simulink model "Antriebsstrangmodell_V2"  (R2019a)
settings: Solver=FixedStepAuto  StartTime=0.0  StopTime=t_Simulation  FixedStep=dt  RelTol=1e-3
undefined symbols (not defined in the file): alpha_Rotor, alpha_Stator, Anteil_Stator, cp_Luft, D_2a, delta, eta_EMaschine_Break_M_EMaschine, eta_EMaschine_Break_M_EMaschine_reku, eta_EMaschine_Break_n_EMaschine, eta_EMaschine_Break_n_EMaschine_reku, eta_EMaschine_Faktor_Volllast, eta_EMaschine_Table, eta_EMaschine_Table_reku, h_WC_pumpoff, h_WC_pumpon, lam_Luft, M_EMaschine_max, m_ER, m_RSL, m_RTO, m_RYO, m_SSL, m_STO, m_SYO, m_WH, nue_Luft, pump_start_limit, rho_Luft, share_EMaschine_Ummagnet_reku_Table, share_EMaschine_Ummagnet_Table, share_EMaschine_Wicklung_reku_Table, share_EMaschine_Wicklung_Table, share_EMaschine_WirkMech_reku_Table, share_EMaschine_WirkMech_Table, share_EMaschine_WirkZus_reku_Table, share_EMaschine_WirkZus_Table, T_Entwurf_Rotor, T_Entwurf_Stator, t_Simulation, T_Start_EMaschine, v_EC_corr, v_ER_corr, v_WH_corr, Verlustleistung_Fit
libraries: fl_lib x72, nesl_utility x26, SimscapeCustomBlocks_lib x8, simulink x3
(part 1 of 2)
settings Model: Creator=Ludwig Stolle  LastModifiedBy=Ludwig Stolle
settings DataIOCC: SaveOutput=off  SignalLogging=off  DSMLogging=off  SaveTime=off  ReturnWorkspaceOutputs=off
settings DebuggingCC: UnconnectedInputMsg=none  UnconnectedOutputMsg=none

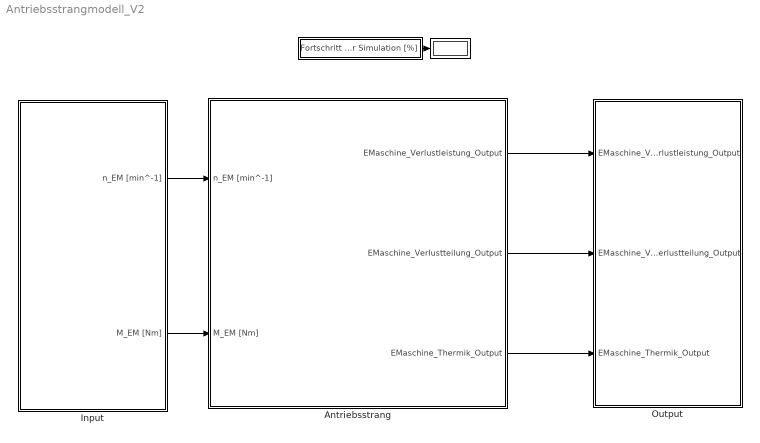
== system Antriebsstrangmodell_V2 ==
  "\t\t     " : Subsystem
  " " : Display
      settings: Format=bank
  Antriebsstrang : Subsystem
  Input : Subsystem
  Output : Subsystem
  wires:
  Input/1(n_EM [min^-1]) -> Antriebsstrang/1(n_EM [min^-1])
  Input/2(M_EM [Nm]) -> Antriebsstrang/2(M_EM [Nm])
  "\t\t     "/1(Fortschritt der Simulation [%]) -> " "/1
  Antriebsstrang/1(EMaschine_Verlustleistung_Output) -> Output/1(EMaschine_Verlustleistung_Output)
  Antriebsstrang/2(EMaschine_Verlustteilung_Output) -> Output/2(EMaschine_Verlustteilung_Output)
  Antriebsstrang/3(EMaschine_Thermik_Output) -> Output/3(EMaschine_Thermik_Output)

== system Antriebsstrangmodell_V2/		      ==
  note: Fortschritt der Simulation = 100 * simulierte Zeit / t_Simulation
      |
      | mit Fortschritt der Simulation in %
  Clock : Clock
  Constant : Constant  Value=t_Simulation  VectorParams1D=off
  Divide : Product  Inputs=*/
  Umrechnung in % : Gain  Gain=100
  Fortschritt der Simulation [%] : Outport
  wires:
  Constant/1 -> Divide/2
  Clock/1 -> Divide/1
  Divide/1 -> Umrechnung in %/1
  Umrechnung in %/1 -> Fortschritt der Simulation [%]/1

== system Antriebsstrangmodell_V2/Antriebsstrang ==
  n_EM [min^-1] : Inport
  M_EM [Nm] : Inport  Port=2
  E-Maschine Thermik : Subsystem
  E-Maschine Verlustleistung : Subsystem
  E-Maschine Verlustteilung : Subsystem
  EMaschine_Verlustleistung_Output : Outport
  EMaschine_Verlustteilung_Output : Outport  Port=2
  EMaschine_Thermik_Output : Outport  Port=3
  wires:
  M_EM [Nm]/1 -> E-Maschine Verlustteilung/3(M_EM [Nm]), E-Maschine Verlustleistung/2(M_EM [Nm])
  n_EM [min^-1]/1 -> E-Maschine Thermik/2(n_EM [min^-1]), E-Maschine Verlustteilung/2(n_EM [min^-1]), E-Maschine Verlustleistung/1(n_EM [min^-1])
  E-Maschine Verlustleistung/1(EMaschine_Verlustleistung_Output) -> EMaschine_Verlustleistung_Output/1, E-Maschine Verlustteilung/1(EMaschine_Verlustleistung_Output)
  E-Maschine Verlustteilung/1(EMaschine_Verlustteilung_Output) -> EMaschine_Verlustteilung_Output/1, E-Maschine Thermik/1(EMaschine_Verlustlteilung_Output)
  E-Maschine Thermik/1(EMaschine_Thermik_Output) -> EMaschine_Thermik_Output/1

== system Antriebsstrangmodell_V2/Input ==
  From Workspace : FromWorkspace  VariableName=n_EM  SampleTime=0  OutputAfterFinalValue=Setting to zero
  From Workspace1 : FromWorkspace  VariableName=M_EM  SampleTime=0  OutputAfterFinalValue=Setting to zero
  Product : Product
  Ramp : simulink/Sources/Ramp  slope=0.05  start=0  InitialOutput=0
  Saturation : Saturate  UpperLimit=1  LowerLimit=0
  n_EM [min^-1] : Outport
  M_EM [Nm] : Outport  Port=2
  wires:
  From Workspace/1 -> n_EM [min^-1]/1
  Saturation/1 -> Product/2
  From Workspace1/1 -> Product/1
  Product/1 -> M_EM [Nm]/1
  Ramp/1 -> Saturation/1

== system Antriebsstrangmodell_V2/Output ==
  note: -> Die Simulationsergebnisse, die an MATLAB übergeben werden sollen, müssen einkommentiert sein
      | -> Falls bestimmte Simualtionsergebnisse nicht an MATLAB übergeben werden sollen, dann müssen diese auskommentiert werden
  EMaschine_Verlustleistung_Output : Inport
  EMaschine_Verlustteilung_Output : Inport  Port=2
  EMaschine_Thermik_Output : Inport  Port=3
  E-Maschine Thermik : ToWorkspace  VariableName=EMaschine_Thermik_Output  SaveFormat=Timeseries  SampleTime=-1
      settings: Decimation=Decimation_Output
  E-Maschine Verlustleistung : ToWorkspace  VariableName=EMaschine_Verlustleistung_Output  SaveFormat=Timeseries  SampleTime=-1
      settings: Decimation=Decimation_Output
  E-Maschine Verlustteilung : ToWorkspace  VariableName=EMaschine_Verlustteilung_Output  SaveFormat=Timeseries  SampleTime=-1
      settings: Decimation=Decimation_Output
  wires:
  EMaschine_Verlustleistung_Output/1 -> E-Maschine Verlustleistung/1
  EMaschine_Verlustteilung_Output/1 -> E-Maschine Verlustteilung/1
  EMaschine_Thermik_Output/1 -> E-Maschine Thermik/1

== system Antriebsstrangmodell_V2/Antriebsstrang/E-Maschine Thermik ==
  EMaschine_Verlustlteilung_Output : Inport
  n_EM [min^-1] : Inport  Port=2
  Aufteilung mechanischer Verluste : Subsystem
  Bus Creator : BusCreator  Inputs=5
  Bus Selector1 : BusSelector  OutputSignals=P_Verlust_EMaschine_Wicklung [W],P_Verlust_EMaschine_Ummagnet [W],P_Verlust_EMaschine_WirkZus [W],P_Verlust_EMaschine_WirkMech [W]
  Thermisches Netzwerk1 : Subsystem
  Wärmeübergangskoeffizienten Konvektion Luftspalt und Endcap-Luft : Subsystem
  EMaschine_Thermik_Output : Outport
  wires:
  EMaschine_Verlustlteilung_Output/1 -> Bus Selector1/1
  Bus Creator/1 -> EMaschine_Thermik_Output/1
  Bus Selector1/2 -> Thermisches Netzwerk1/2(P_Verlust_EMaschine_Ummagnet [W])  "<P_Verlust_EMaschine_Ummagnet [W]>"
  Bus Selector1/3 -> Thermisches Netzwerk1/3(P_Verlust_EMaschine_WirkZus [W])  "<P_Verlust_EMaschine_WirkZus [W]>"
  Bus Selector1/1 -> Thermisches Netzwerk1/1(P_Verlust_EMaschine_Wicklung [W])  "<P_Verlust_EMaschine_Wicklung [W]>"
  Wärmeübergangskoeffizienten Konvektion Luftspalt und Endcap-Luft/1(HTC_Luftspalt [W*m^-2*K^-1]) -> Thermisches Netzwerk1/6(HTC_Luftspalt [W*m^-2*K^-1])  "HTC_Luftspalt [W*m^-2*K^-1]"
  Wärmeübergangskoeffizienten Konvektion Luftspalt und Endcap-Luft/2(HTC_Endcap [W*m^-2*K^-1]) -> Thermisches Netzwerk1/7(HTC_Endcap [W*m^-2*K^-1])  "HTC_Endcap [W*m^-2*K^-1]"
  Wärmeübergangskoeffizienten Konvektion Luftspalt und Endcap-Luft/3(HTC_Kurzschlussring [W*m^-2*K^-1]) -> Thermisches Netzwerk1/8(HTC_Kurzschlussring [W*m^-2*K^-1])  "HTC_Kurzschlussring [W*m^-2*K^-1]"
  Wärmeübergangskoeffizienten Konvektion Luftspalt und Endcap-Luft/4(HTC_Wickelkopf [W*m^-2*K^-1]) -> Thermisches Netzwerk1/9(HTC_Wickelkopf [W*m^-2*K^-1])  "HTC_Wickelkopf [W*m^-2*K^-1]"
  Aufteilung mechanischer Verluste/1(P_Verlust_EMaschine_Luftwiderstand [W]) -> Thermisches Netzwerk1/4(P_Verlust_EMaschine_Luftwiderstand [W])
  Bus Selector1/4 -> Aufteilung mechanischer Verluste/1(P_Verlust_EMaschine_WirkMech [W])  "<P_Verlust_EMaschine_WirkMech [W]>"
  Aufteilung mechanischer Verluste/2(P_Verlust_EMaschine_Lager [W]) -> Thermisches Netzwerk1/5(P_Verlust_EMaschine_Lager [W])
  Thermisches Netzwerk1/1(T_EMaschine_Wickelkopf [K]) -> Bus Creator/1
  Thermisches Netzwerk1/2(T_EMaschine_Kuehlmittel [K]) -> Bus Creator/2
  n_EM [min^-1]/1 -> Aufteilung mechanischer Verluste/2(n_EMaschine [min^-1]), Wärmeübergangskoeffizienten Konvektion Luftspalt und Endcap-Luft/1(<n_EMaschine [min^-1]>)
  Thermisches Netzwerk1/4(T_EMaschine_Kurzschlussring [K]) -> Bus Creator/4
  Thermisches Netzwerk1/5(T_EMaschine_Rotorstaebe [K]) -> Bus Creator/5
  Thermisches Netzwerk1/3(T_EMaschine_Wicklung [K]) -> Bus Creator/3

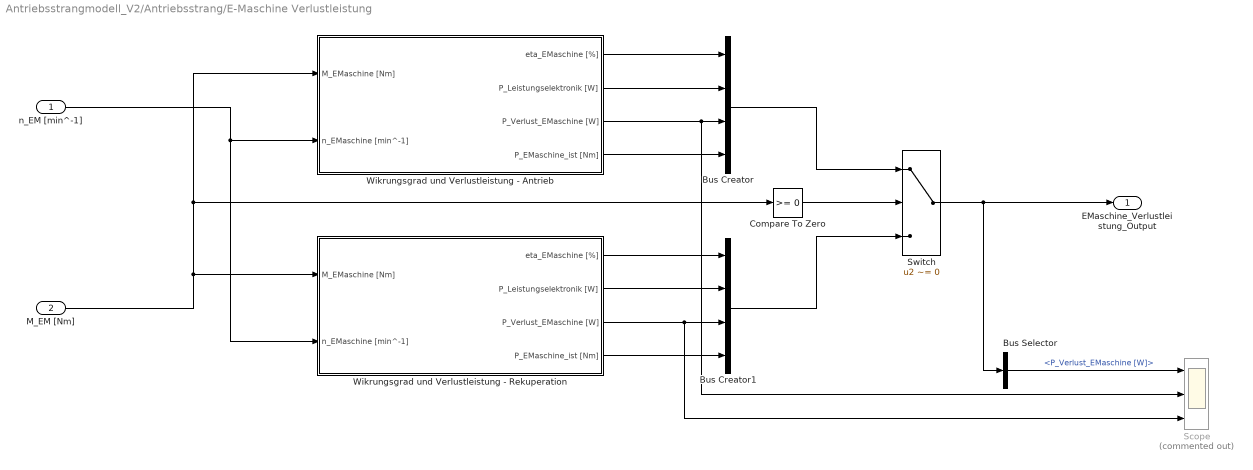
== system Antriebsstrangmodell_V2/Antriebsstrang/E-Maschine Verlustleistung ==
  n_EM [min^-1] : Inport
  M_EM [Nm] : Inport  Port=2
  Bus Creator : BusCreator  Inputs=4
  Bus Creator1 : BusCreator  Inputs=4
  Bus Selector : BusSelector  OutputSignals=P_Verlust_EMaschine [W]
  Compare To Zero : simulink/Logic and Bit Operations/Compare To Zero  relop=>=  OutDataTypeStr=boolean
  Scope : Scope  Commented=on  NumInputPorts=3
  Switch : Switch  Criteria=u2 ~= 0
  Wikrungsgrad und Verlustleistung - Antrieb : Subsystem
  Wikrungsgrad und Verlustleistung - Rekuperation : Subsystem
  EMaschine_Verlustleistung_Output : Outport
  wires:
  Wikrungsgrad und Verlustleistung - Antrieb/1(eta_EMaschine [%]) -> Bus Creator/1
  Wikrungsgrad und Verlustleistung - Antrieb/2(P_Leistungselektronik [W]) -> Bus Creator/2
  Wikrungsgrad und Verlustleistung - Antrieb/3(P_Verlust_EMaschine [W]) -> Scope/2, Bus Creator/3
  Wikrungsgrad und Verlustleistung - Rekuperation/1(eta_EMaschine [%]) -> Bus Creator1/1
  Wikrungsgrad und Verlustleistung - Rekuperation/2(P_Leistungselektronik [W]) -> Bus Creator1/2
  Wikrungsgrad und Verlustleistung - Rekuperation/3(P_Verlust_EMaschine [W]) -> Scope/3, Bus Creator1/3
  Bus Creator/1 -> Switch/1
  Bus Creator1/1 -> Switch/3
  Compare To Zero/1 -> Switch/2
  Switch/1 -> Bus Selector/1, EMaschine_Verlustleistung_Output/1
  Bus Selector/1 -> Scope/1  "<P_Verlust_EMaschine [W]>"
  Wikrungsgrad und Verlustleistung - Antrieb/4(P_EMaschine_ist [Nm]) -> Bus Creator/4
  Wikrungsgrad und Verlustleistung - Rekuperation/4(P_EMaschine_ist [Nm]) -> Bus Creator1/4
  n_EM [min^-1]/1 -> Wikrungsgrad und Verlustleistung - Rekuperation/2(n_EMaschine [min^-1]), Wikrungsgrad und Verlustleistung - Antrieb/2(n_EMaschine [min^-1])
  M_EM [Nm]/1 -> Wikrungsgrad und Verlustleistung - Antrieb/1(M_EMaschine [Nm]), Compare To Zero/1, Wikrungsgrad und Verlustleistung - Rekuperation/1(M_EMaschine [Nm])

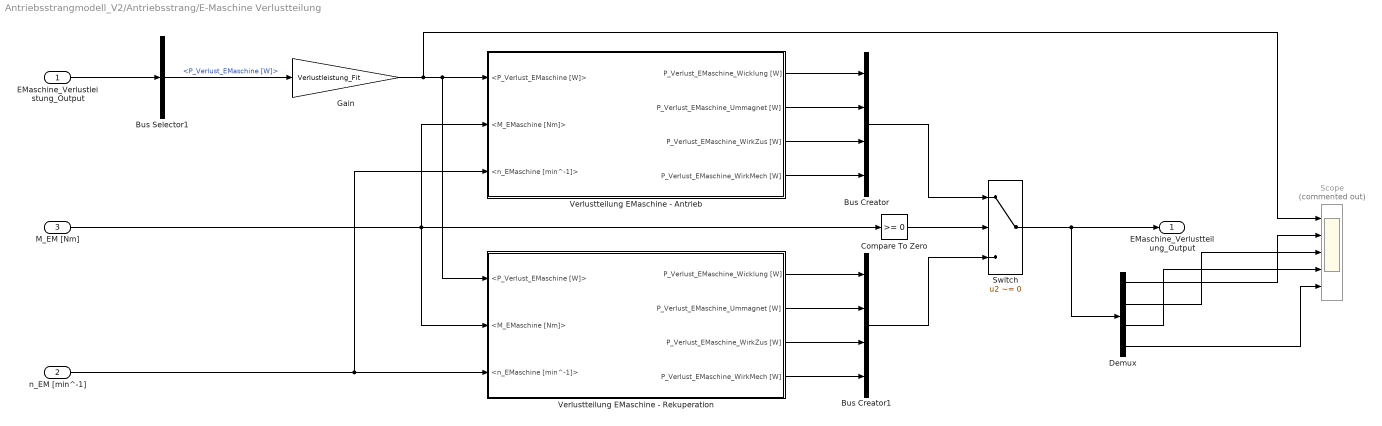
== system Antriebsstrangmodell_V2/Antriebsstrang/E-Maschine Verlustteilung ==
  EMaschine_Verlustleistung_Output : Inport
  n_EM [min^-1] : Inport  Port=2
  M_EM [Nm] : Inport  Port=3
  Bus Creator : BusCreator  Inputs=4
  Bus Creator1 : BusCreator  Inputs=4
  Bus Selector1 : BusSelector  OutputSignals=P_Verlust_EMaschine [W]
  Compare To Zero : simulink/Logic and Bit Operations/Compare To Zero  relop=>=  OutDataTypeStr=boolean
  Demux : Demux
  Gain : Gain  Gain=Verlustleistung_Fit
  Scope : Scope  Commented=on  NumInputPorts=5
  Switch : Switch  Criteria=u2 ~= 0
  Verlustteilung EMaschine - Antrieb : Subsystem
  Verlustteilung EMaschine - Rekuperation : Subsystem
  EMaschine_Verlustteilung_Output : Outport
  wires:
  EMaschine_Verlustleistung_Output/1 -> Bus Selector1/1
  Bus Selector1/1 -> Gain/1  "<P_Verlust_EMaschine [W]>"
  Verlustteilung EMaschine - Antrieb/1(P_Verlust_EMaschine_Wicklung [W]) -> Bus Creator/1
  Verlustteilung EMaschine - Antrieb/2(P_Verlust_EMaschine_Ummagnet [W]) -> Bus Creator/2
  Verlustteilung EMaschine - Antrieb/3(P_Verlust_EMaschine_WirkZus [W]) -> Bus Creator/3
  Verlustteilung EMaschine - Antrieb/4(P_Verlust_EMaschine_WirkMech [W]) -> Bus Creator/4
  Compare To Zero/1 -> Switch/2
  Switch/1 -> Demux/1, EMaschine_Verlustteilung_Output/1
  Bus Creator/1 -> Switch/1
  Verlustteilung EMaschine - Rekuperation/1(P_Verlust_EMaschine_Wicklung [W]) -> Bus Creator1/1
  Verlustteilung EMaschine - Rekuperation/2(P_Verlust_EMaschine_Ummagnet [W]) -> Bus Creator1/2
  Verlustteilung EMaschine - Rekuperation/3(P_Verlust_EMaschine_WirkZus [W]) -> Bus Creator1/3
  Verlustteilung EMaschine - Rekuperation/4(P_Verlust_EMaschine_WirkMech [W]) -> Bus Creator1/4
  Bus Creator1/1 -> Switch/3
  Gain/1 -> Scope/1, Verlustteilung EMaschine - Rekuperation/1(<P_Verlust_EMaschine [W]>), Verlustteilung EMaschine - Antrieb/1(<P_Verlust_EMaschine [W]>)
  Demux/4 -> Scope/5
  Demux/1 -> Scope/2
  Demux/2 -> Scope/3
  Demux/3 -> Scope/4
  n_EM [min^-1]/1 -> Verlustteilung EMaschine - Antrieb/3(<n_EMaschine [min^-1]>), Verlustteilung EMaschine - Rekuperation/3(<n_EMaschine [min^-1]>)
  M_EM [Nm]/1 -> Verlustteilung EMaschine - Rekuperation/2(<M_EMaschine [Nm]>), Verlustteilung EMaschine - Antrieb/2(<M_EMaschine [Nm]>), Compare To Zero/1

== system Antriebsstrangmodell_V2/Antriebsstrang/E-Maschine Thermik/Aufteilung mechanischer Verluste ==
  note: Berechnung der Anteile von Luftwiderstand und Lagerverlusten an ges. mechanischem Verlust nach CHIN 2018.
      | Verluste sind nur von der Drehzahl abhängig. Daher normierte Verluste angenähert mittels Polynom 2. Grades für Luftwiderstand
      | und Polynom 1. Grades für Lagerreibung.
  P_Verlust_EMaschine_WirkMech [W] : Inport
  n_EMaschine [min^-1] : Inport  Port=2
  Abs : Abs
  Add : Sum
  Add1 : Sum  Inputs=+-
  Divide : Product  Inputs=/*
  Divide1 : Product  Inputs=**
  Polynomial : Polyval  Coefs=[+0.0026e-5, -0.25e-5, 0]
  Polynomial1 : Polyval  Coefs=[+0.06e-3, +0.05]
  P_Verlust_EMaschine_Luftwiderstand [W] : Outport
  P_Verlust_EMaschine_Lager [W] : Outport  Port=2
  wires:
  n_EMaschine [min^-1]/1 -> Abs/1
  Abs/1 -> Polynomial1/1, Polynomial/1
  Polynomial1/1 -> Divide/2, Add/2  "Normierter Lagerverlust"
  Polynomial/1 -> Add/1  "Normierte Luftreibung"
  Add/1 -> Divide/1
  P_Verlust_EMaschine_WirkMech [W]/1 -> Add1/1, Divide1/1
  Divide/1 -> Divide1/2  "Anteil Lagerverluste am gesamten mechanischen Verlust"
  Divide1/1 -> Add1/2, P_Verlust_EMaschine_Lager [W]/1  "P_Verlust_EMaschine_Lager [W]"
  Add1/1 -> P_Verlust_EMaschine_Luftwiderstand [W]/1  "P_Verlust_EMaschine_Luftwiderstand [W]"

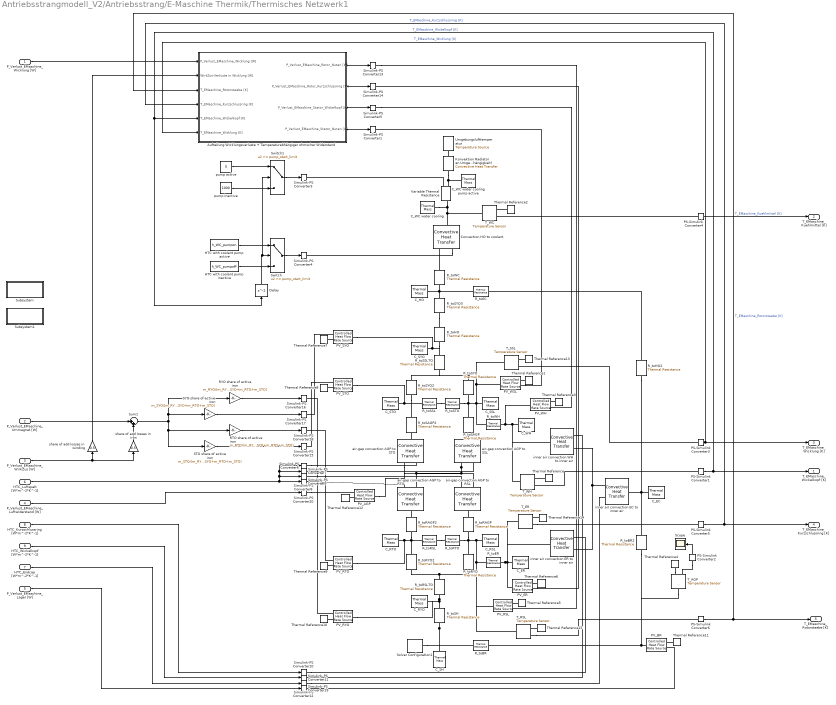
== system Antriebsstrangmodell_V2/Antriebsstrang/E-Maschine Thermik/Thermisches Netzwerk1 ==
  P_Verlust_EMaschine_Wicklung [W] : Inport
  P_Verlust_EMaschine_Ummagnet [W] : Inport  Port=2
  P_Verlust_EMaschine_WirkZus [W] : Inport  Port=3
  P_Verlust_EMaschine_Luftwiderstand [W] : Inport  Port=4
  P_Verlust_EMaschine_Lager [W] : Inport  Port=5
  HTC_Luftspalt [W*m^-2*K^-1] : Inport  Port=6
  HTC_Endcap [W*m^-2*K^-1] : Inport  Port=7
  HTC_Kurzschlussring [W*m^-2*K^-1] : Inport  Port=8
  HTC_Wickelkopf [W*m^-2*K^-1] : Inport  Port=9
  Aufteilung Wicklungsverluste + Temperaturabhängiger ohmscher Widerstand : Subsystem
  C_EC : fl_lib/Thermal/Thermal Elements/Thermal Mass  mass=m_EC kg  sp_heat=cp_EC J/kg/K  T_specify=on  T_priority=High  T=T_Start_EMaschine K  T_nominal_specify=off  T_nominal_unit=K  T_nominal_value=1  Q_specify=off  Q_priority=None  Q=0 W  Q_nominal_specify=off  Q_nominal_unit=W  Q_nominal_value=1
  C_ER : fl_lib/Thermal/Thermal Elements/Thermal Mass  mass=m_ER kg  sp_heat=cp_ER J/kg/K  T_specify=on  T_priority=High  T=T_Start_EMaschine K  T_nominal_specify=off  T_nominal_unit=K  T_nominal_value=1  Q_specify=off  Q_priority=None  Q=0 W  Q_nominal_specify=off  Q_nominal_unit=W  Q_nominal_value=1
  C_HO : fl_lib/Thermal/Thermal Elements/Thermal Mass  mass=m_HO kg  sp_heat=cp_HO J/kg/K  T_specify=on  T_priority=High  T=T_Start_EMaschine K  T_nominal_specify=off  T_nominal_unit=K  T_nominal_value=1  Q_specify=off  Q_priority=None  Q=0 W  Q_nominal_specify=off  Q_nominal_unit=W  Q_nominal_value=1
  C_RSL : fl_lib/Thermal/Thermal Elements/Thermal Mass  mass=m_RSL kg  sp_heat=cp_RSL J/kg/K  T_specify=on  T_priority=High  T=T_Start_EMaschine K  T_nominal_specify=off  T_nominal_unit=K  T_nominal_value=1  Q_specify=off  Q_priority=None  Q=0 W  Q_nominal_specify=off  Q_nominal_unit=W  Q_nominal_value=1
  C_RTO : fl_lib/Thermal/Thermal Elements/Thermal Mass  mass=m_RTO kg  sp_heat=cp_RTO J/kg/K  T_specify=on  T_priority=High  T=T_Start_EMaschine K  T_nominal_specify=off  T_nominal_unit=K  T_nominal_value=1  Q_specify=off  Q_priority=None  Q=0 W  Q_nominal_specify=off  Q_nominal_unit=W  Q_nominal_value=1
  C_RYO : fl_lib/Thermal/Thermal Elements/Thermal Mass  mass=m_RYO kg  sp_heat=cp_RYO J/kg/K  T_specify=on  T_priority=High  T=T_Start_EMaschine K  T_nominal_specify=off  T_nominal_unit=K  T_nominal_value=1  Q_specify=off  Q_priority=None  Q=0 W  Q_nominal_specify=off  Q_nominal_unit=W  Q_nominal_value=1
  C_SH : fl_lib/Thermal/Thermal Elements/Thermal Mass  mass=m_SH kg  sp_heat=cp_SH J/kg/K  T_specify=on  T_priority=High  T=T_Start_EMaschine K  T_nominal_specify=off  T_nominal_unit=K  T_nominal_value=1  Q_specify=off  Q_priority=None  Q=0 W  Q_nominal_specify=off  Q_nominal_unit=W  Q_nominal_value=1
  C_SSL : fl_lib/Thermal/Thermal Elements/Thermal Mass  mass=m_SSL kg  sp_heat=cp_SSL J/kg/K  T_specify=on  T_priority=High  T=T_Start_EMaschine K  T_nominal_specify=off  T_nominal_unit=K  T_nominal_value=1  Q_specify=off  Q_priority=None  Q=0 W  Q_nominal_specify=off  Q_nominal_unit=W  Q_nominal_value=1
  C_STO : fl_lib/Thermal/Thermal Elements/Thermal Mass  mass=m_STO kg  sp_heat=cp_STO J/kg/K  T_specify=on  T_priority=High  T=T_Start_EMaschine K  T_nominal_specify=off  T_nominal_unit=K  T_nominal_value=1  Q_specify=off  Q_priority=None  Q=0 W  Q_nominal_specify=off  Q_nominal_unit=W  Q_nominal_value=1
  C_SYO : fl_lib/Thermal/Thermal Elements/Thermal Mass  mass=m_SYO kg  sp_heat=cp_SYO J/kg/K  T_specify=on  T_priority=High  T=T_Start_EMaschine K  T_nominal_specify=off  T_nominal_unit=K  T_nominal_value=1  Q_specify=off  Q_priority=None  Q=0 W  Q_nominal_specify=off  Q_nominal_unit=W  Q_nominal_value=1
  C_WC water cooling : fl_lib/Thermal/Thermal Elements/Thermal Mass  mass=m_WC kg  sp_heat=cp_WC J/kg/K  T_specify=on  T_priority=High  T=T_Start_EMaschine K  T_nominal_specify=off  T_nominal_unit=K  T_nominal_value=1  Q_specify=off  Q_priority=None  Q=0 W  Q_nominal_specify=off  Q_nominal_unit=W  Q_nominal_value=1
  C_WC water cooling pump active : fl_lib/Thermal/Thermal Elements/Thermal Mass  mass=m_WC_pumpon kg  sp_heat=cp_WC J/kg/K  T_specify=on  T_priority=High  T=T_Start_EMaschine K  T_nominal_specify=off  T_nominal_unit=K  T_nominal_value=1  Q_specify=off  Q_priority=None  Q=0 W  Q_nominal_specify=off  Q_nominal_unit=W  Q_nominal_value=1
  C_WH : fl_lib/Thermal/Thermal Elements/Thermal Mass  mass=m_WH kg  sp_heat=cp_WH J/kg/K  T_specify=on  T_priority=High  T=T_Start_EMaschine K  T_nominal_specify=off  T_nominal_unit=K  T_nominal_value=1  Q_specify=off  Q_priority=None  Q=0 W  Q_nominal_specify=off  Q_nominal_unit=W  Q_nominal_value=1
  Convection HO to coolant : SimscapeCustomBlocks_lib/Convective Heat Transfer  area=A_HO m^2  T_specify=off  T_priority=None  T=0 K  T_nominal_specify=off  T_nominal_unit=K  T_nominal_value=1  Q_specify=off  Q_priority=None  Q=0 W  Q_nominal_specify=off  Q_nominal_unit=W  Q_nominal_value=1
  Delay : Delay
  HTC with coolant pump active : Constant  Value=h_WC_pumpon
  HTC with coolant pump inactive : Constant  Value=h_WC_pumpoff
  Konvektion Radiator an Umgebungsluft (keine Geschw.Abhängigkeit) : fl_lib/Thermal/Thermal Elements/Convective Heat Transfer  area=1 m^2  heat_tr_coeff=radiator_power W/(m^2 * K)  T_specify=off  T_priority=None  T=0 K  T_nominal_specify=off  T_nominal_unit=K  T_nominal_value=1  Q_specify=off  Q_priority=None  Q=0 W  Q_nominal_specify=off  Q_nominal_unit=W  Q_nominal_value=1
  PS-Simulink Converter{1..6} (6 alike) : nesl_utility/PS-Simulink Converter  PhysicalDomain=network_engine_domain  SubClassName=ps_output  LeftPortType=input  RightPortType=output  PseudoPeriodic=off  Frequencies=[]  Unit=1  AffineConversion=off
  PV_AGP : fl_lib/Thermal/Thermal Sources/Controlled Heat Flow Rate Source
      settings: SourceProductName=Simscape
  PV_BR : fl_lib/Thermal/Thermal Sources/Controlled Heat Flow Rate Source
      settings: SourceProductName=Simscape
  PV_ER : fl_lib/Thermal/Thermal Sources/Controlled Heat Flow Rate Source
      settings: SourceProductName=Simscape
  PV_RSL : fl_lib/Thermal/Thermal Sources/Controlled Heat Flow Rate Source
      settings: SourceProductName=Simscape
  PV_RTO : fl_lib/Thermal/Thermal Sources/Controlled Heat Flow Rate Source
      settings: SourceProductName=Simscape
  PV_RYO : fl_lib/Thermal/Thermal Sources/Controlled Heat Flow Rate Source
      settings: SourceProductName=Simscape
  PV_STO : fl_lib/Thermal/Thermal Sources/Controlled Heat Flow Rate Source
      settings: SourceProductName=Simscape
  PV_SYO : fl_lib/Thermal/Thermal Sources/Controlled Heat Flow Rate Source
      settings: SourceProductName=Simscape
  PV_WH : fl_lib/Thermal/Thermal Sources/Controlled Heat Flow Rate Source
      settings: SourceProductName=Simscape
  PV_WSL : fl_lib/Thermal/Thermal Sources/Controlled Heat Flow Rate Source
      settings: SourceProductName=Simscape
  RTO share of active iron : Gain  Gain=m_RTO/(m_RYO+m_SYO+m_RTO+m_STO)
  RYO share of active iron : Gain  Gain=m_RYO/(m_RYO+m_SYO+m_RTO+m_STO)
  R_toBR : fl_lib/Thermal/Thermal Elements/Thermal Resistance  resistance=R_toBR K/W  T_specify=off  T_priority=None  T=0 K  T_nominal_specify=off  T_nominal_unit=K  T_nominal_value=1  Q_specify=off  Q_priority=None  Q=0 W  Q_nominal_specify=off  Q_nominal_unit=W  Q_nominal_value=1
      settings: SourceProductName=Simscape  SourceProductBaseCode=SS
  R_toBR2 : fl_lib/Thermal/Thermal Elements/Thermal Resistance  resistance=R_toBR2 K/W  T_specify=off  T_priority=None  T=0 K  T_nominal_specify=off  T_nominal_unit=K  T_nominal_value=1  Q_specify=off  Q_priority=None  Q=0 W  Q_nominal_specify=off  Q_nominal_unit=W  Q_nominal_value=1
      settings: SourceProductName=Simscape  SourceProductBaseCode=SS
  R_toEC : fl_lib/Thermal/Thermal Elements/Thermal Resistance  resistance=R_toEC K/W  T_specify=off  T_priority=None  T=0 K  T_nominal_specify=off  T_nominal_unit=K  T_nominal_value=1  Q_specify=off  Q_priority=None  Q=0 W  Q_nominal_specify=off  Q_nominal_unit=W  Q_nominal_value=1
      settings: SourceProductName=Simscape  SourceProductBaseCode=SS
  R_toER : fl_lib/Thermal/Thermal Elements/Thermal Resistance  resistance=R_toER K/W  T_specify=off  T_priority=None  T=0 K  T_nominal_specify=off  T_nominal_unit=K  T_nominal_value=1  Q_specify=off  Q_priority=None  Q=0 W  Q_nominal_specify=off  Q_nominal_unit=W  Q_nominal_value=1
      settings: SourceProductName=Simscape  SourceProductBaseCode=SS
  R_toHO : fl_lib/Thermal/Thermal Elements/Thermal Resistance  resistance=R_toHO K/W  T_specify=off  T_priority=None  T=0 K  T_nominal_specify=off  T_nominal_unit=K  T_nominal_value=1  Q_specify=off  Q_priority=None  Q=0 W  Q_nominal_specify=off  Q_nominal_unit=W  Q_nominal_value=1
      settings: SourceProductName=Simscape  SourceProductBaseCode=SS
  R_toHO2 : fl_lib/Thermal/Thermal Elements/Thermal Resistance  resistance=R_toHO2 K/W  T_specify=off  T_priority=None  T=0 K  T_nominal_specify=off  T_nominal_unit=K  T_nominal_value=1  Q_specify=off  Q_priority=None  Q=0 W  Q_nominal_specify=off  Q_nominal_unit=W  Q_nominal_value=1
      settings: SourceProductName=Simscape  SourceProductBaseCode=SS
  R_toRAGP : fl_lib/Thermal/Thermal Elements/Thermal Resistance  resistance=R_toRAGP K/W  T_specify=off  T_priority=None  T=0 K  T_nominal_specify=off  T_nominal_unit=K  T_nominal_value=1  Q_specify=off  Q_priority=None  Q=0 W  Q_nominal_specify=off  Q_nominal_unit=W  Q_nominal_value=1
      settings: SourceProductName=Simscape  SourceProductBaseCode=SS
  R_toRAGP2 : fl_lib/Thermal/Thermal Elements/Thermal Resistance  resistance=R_toRAGP2 K/W  T_specify=off  T_priority=None  T=0 K  T_nominal_specify=off  T_nominal_unit=K  T_nominal_value=1  Q_specify=off  Q_priority=None  Q=0 W  Q_nominal_specify=off  Q_nominal_unit=W  Q_nominal_value=1
      settings: SourceProductName=Simscape  SourceProductBaseCode=SS
  R_toRSL : fl_lib/Thermal/Thermal Elements/Thermal Resistance  resistance=R_toRSL K/W  T_specify=off  T_priority=None  T=0 K  T_nominal_specify=off  T_nominal_unit=K  T_nominal_value=1  Q_specify=off  Q_priority=None  Q=0 W  Q_nominal_specify=off  Q_nominal_unit=W  Q_nominal_value=1
      settings: SourceProductName=Simscape  SourceProductBaseCode=SS
  R_toRSLTO : fl_lib/Thermal/Thermal Elements/Thermal Resistance  resistance=R_toRSLTO K/W  T_specify=off  T_priority=None  T=0 K  T_nominal_specify=off  T_nominal_unit=K  T_nominal_value=1  Q_specify=off  Q_priority=None  Q=0 W  Q_nominal_specify=off  Q_nominal_unit=W  Q_nominal_value=1
      settings: SourceProductName=Simscape  SourceProductBaseCode=SS
  R_toRTO : fl_lib/Thermal/Thermal Elements/Thermal Resistance  resistance=R_toRTO K/W  T_specify=off  T_priority=None  T=0 K  T_nominal_specify=off  T_nominal_unit=K  T_nominal_value=1  Q_specify=off  Q_priority=None  Q=0 W  Q_nominal_specify=off  Q_nominal_unit=W  Q_nominal_value=1
      settings: SourceProductName=Simscape  SourceProductBaseCode=SS
  R_toRYO : fl_lib/Thermal/Thermal Elements/Thermal Resistance  resistance=R_toRYO K/W  T_specify=off  T_priority=None  T=0 K  T_nominal_specify=off  T_nominal_unit=K  T_nominal_value=1  Q_specify=off  Q_priority=None  Q=0 W  Q_nominal_specify=off  Q_nominal_unit=W  Q_nominal_value=1
      settings: SourceProductName=Simscape  SourceProductBaseCode=SS
  R_toRYO2 : fl_lib/Thermal/Thermal Elements/Thermal Resistance  resistance=R_toRYO2 K/W  T_specify=off  T_priority=None  T=0 K  T_nominal_specify=off  T_nominal_unit=K  T_nominal_value=1  Q_specify=off  Q_priority=None  Q=0 W  Q_nominal_specify=off  Q_nominal_unit=W  Q_nominal_value=1
      settings: SourceProductName=Simscape  SourceProductBaseCode=SS
  R_toSAGP : fl_lib/Thermal/Thermal Elements/Thermal Resistance  resistance=R_toSAGP K/W  T_specify=off  T_priority=None  T=0 K  T_nominal_specify=off  T_nominal_unit=K  T_nominal_value=1  Q_specify=off  Q_priority=None  Q=0 W  Q_nominal_specify=off  Q_nominal_unit=W  Q_nominal_value=1
      settings: SourceProductName=Simscape  SourceProductBaseCode=SS
  R_toSAGP2 : fl_lib/Thermal/Thermal Elements/Thermal Resistance  resistance=R_toSAGP2 K/W  T_specify=off  T_priority=None  T=0 K  T_nominal_specify=off  T_nominal_unit=K  T_nominal_value=1  Q_specify=off  Q_priority=None  Q=0 W  Q_nominal_specify=off  Q_nominal_unit=W  Q_nominal_value=1
      settings: SourceProductName=Simscape  SourceProductBaseCode=SS
  R_toSH : fl_lib/Thermal/Thermal Elements/Thermal Resistance  resistance=R_toSH K/W  T_specify=off  T_priority=None  T=0 K  T_nominal_specify=off  T_nominal_unit=K  T_nominal_value=1  Q_specify=off  Q_priority=None  Q=0 W  Q_nominal_specify=off  Q_nominal_unit=W  Q_nominal_value=1
      settings: SourceProductName=Simscape  SourceProductBaseCode=SS
  R_toSSL : fl_lib/Thermal/Thermal Elements/Thermal Resistance  resistance=R_toSSL K/W  T_specify=off  T_priority=None  T=0 K  T_nominal_specify=off  T_nominal_unit=K  T_nominal_value=1  Q_specify=off  Q_priority=None  Q=0 W  Q_nominal_specify=off  Q_nominal_unit=W  Q_nominal_value=1
      settings: SourceProductName=Simscape  SourceProductBaseCode=SS
  R_toSSLTO : fl_lib/Thermal/Thermal Elements/Thermal Resistance  resistance=R_toSSLTO K/W  T_specify=off  T_priority=None  T=0 K  T_nominal_specify=off  T_nominal_unit=K  T_nominal_value=1  Q_specify=off  Q_priority=None  Q=0 W  Q_nominal_specify=off  Q_nominal_unit=W  Q_nominal_value=1
      settings: SourceProductName=Simscape  SourceProductBaseCode=SS
  R_toSTO : fl_lib/Thermal/Thermal Elements/Thermal Resistance  resistance=R_toSTO K/W  T_specify=off  T_priority=None  T=0 K  T_nominal_specify=off  T_nominal_unit=K  T_nominal_value=1  Q_specify=off  Q_priority=None  Q=0 W  Q_nominal_specify=off  Q_nominal_unit=W  Q_nominal_value=1
      settings: SourceProductName=Simscape  SourceProductBaseCode=SS
  R_toSYO : fl_lib/Thermal/Thermal Elements/Thermal Resistance  resistance=R_toSYO K/W  T_specify=off  T_priority=None  T=0 K  T_nominal_specify=off  T_nominal_unit=K  T_nominal_value=1  Q_specify=off  Q_priority=None  Q=0 W  Q_nominal_specify=off  Q_nominal_unit=W  Q_nominal_value=1
      settings: SourceProductName=Simscape  SourceProductBaseCode=SS
  R_toSYO2 : fl_lib/Thermal/Thermal Elements/Thermal Resistance  resistance=R_toSYO2 K/W  T_specify=off  T_priority=None  T=0 K  T_nominal_specify=off  T_nominal_unit=K  T_nominal_value=1  Q_specify=off  Q_priority=None  Q=0 W  Q_nominal_specify=off  Q_nominal_unit=W  Q_nominal_value=1
      settings: SourceProductName=Simscape  SourceProductBaseCode=SS
  R_toSYO3 : fl_lib/Thermal/Thermal Elements/Thermal Resistance  resistance=R_toSYO3 K/W  T_specify=off  T_priority=None  T=0 K  T_nominal_specify=off  T_nominal_unit=K  T_nominal_value=1  Q_specify=off  Q_priority=None  Q=0 W  Q_nominal_specify=off  Q_nominal_unit=W  Q_nominal_value=1
      settings: SourceProductName=Simscape  SourceProductBaseCode=SS
  R_toWC : fl_lib/Thermal/Thermal Elements/Thermal Resistance  resistance=R_toWC K/W  T_specify=off  T_priority=None  T=0 K  T_nominal_specify=off  T_nominal_unit=K  T_nominal_value=1  Q_specify=off  Q_priority=None  Q=0 W  Q_nominal_specify=off  Q_nominal_unit=W  Q_nominal_value=1
      settings: SourceProductName=Simscape  SourceProductBaseCode=SS
  R_toWH : fl_lib/Thermal/Thermal Elements/Thermal Resistance  resistance=R_toWH K/W  T_specify=off  T_priority=None  T=0 K  T_nominal_specify=off  T_nominal_unit=K  T_nominal_value=1  Q_specify=off  Q_priority=None  Q=0 W  Q_nominal_specify=off  Q_nominal_unit=W  Q_nominal_value=1
      settings: SourceProductName=Simscape  SourceProductBaseCode=SS
  STO share of active iron : Gain  Gain=m_STO/(m_RYO+m_SYO+m_RTO+m_STO)
  SYO share of active iron : Gain  Gain=m_SYO/(m_RYO+m_SYO+m_RTO+m_STO)
  Scope : Scope
  Simulink-PS Converter{1,3..20} (19 alike) : nesl_utility/Simulink-PS Converter  PhysicalDomain=network_engine_domain  SubClassName=ps_input  LeftPortType=input  RightPortType=output  PseudoPeriodic=off  Frequencies=[]  NoiseDistribution=none  NoiseParameters=[]  Unit=1  AffineConversion=off  FilteringAndDerivatives=provide  SimscapeFilterOrder=1  InputFilterTimeConstant=0.001  UdotUserProvided=0
  Solver Configuration1 : nesl_utility/Solver Configuration  PhysicalDomain=network_engine_domain  SubClassName=solver  LeftPortType=input  RightPortType=generic  Tones=[]  Harmonics=[]  SimulateNoise=off  Profile=off  UseLocalSampling=off  EnableSwitchedLinearOptims=on  FrequencyDomain=off  UseCCode=off  RelTol=0.001  AbsTol=1e-06  MinStep=1e-09  ToWorkspace=off  RevertToSquareIcSolve=off  NumHomotopyIterations=100  PhasorMode=off  PhasorModeNumHarmonics=1  DoDC=off  ResidualTolerance=1e-09  UseLocalSolver=on  LocalSolverChoice=NE_BACKWARD_EULER_ADVANCER  LocalSolverSampleTime=dt  DoFixedCost=on  MaxNonlinIter=3  MaxModeIter=2  LinearAlgebra=auto  EquationFormulation=NE_TIME_EF  DelaysMemoryBudget=1024  AutomaticFiltering=on  FilteringTimeConstant=0.001  PartitionStorageMethod=AS_NEEDED  PartitionMemoryBudget=1024  PartitionMethod=FAST
  Subsystem : Subsystem
      settings: OpenFcn=open_system('simscape')
      mask Display: disp(sprintf('Open Simscape\nLibrary'));
  Subsystem1 : Subsystem
      settings: OpenFcn=|
      | load_system('fl_lib');
      | open_system('fl_lib/Thermal');
      mask Display: disp(sprintf('Open Thermal\nLibrary'));
  Sum1 : Sum  Inputs=|++
  Switch : Switch  Threshold=pump_start_limit
  Switch1 : Switch  Threshold=pump_start_limit
  T_AGP : fl_lib/Thermal/Thermal Sensors/Temperature Sensor
  T_ER : fl_lib/Thermal/Thermal Sensors/Temperature Sensor
  T_RSL : fl_lib/Thermal/Thermal Sensors/Temperature Sensor
  T_SSL : fl_lib/Thermal/Thermal Sensors/Temperature Sensor
  T_WC : fl_lib/Thermal/Thermal Sensors/Temperature Sensor
  T_WH : fl_lib/Thermal/Thermal Sensors/Temperature Sensor
  Thermal Reference{,1..15} (16 alike) : fl_lib/Thermal/Thermal Elements/Thermal Reference
  Umgebungslufttemperatur : fl_lib/Thermal/Thermal Sources/Temperature Source  temperature=T_Umgebung K
      settings: SourceProductName=Simscape
  Variable Thermal Resistance : fl_lib/Thermal/Thermal Elements/Variable Thermal Resistance  R_min=0 K/W  T_specify=off  T_priority=None  T=0 K  T_nominal_specify=off  T_nominal_unit=K  T_nominal_value=1  Q_specify=off  Q_priority=None  Q=0 W  Q_nominal_specify=off  Q_nominal_unit=W  Q_nominal_value=1
      settings: SourceProductName=Simscape  SourceProductBaseCode=SS
  air-gap convection AGP to RSL : SimscapeCustomBlocks_lib/Convective Heat Transfer  area=A_RSL m^2  T_specify=off  T_priority=None  T=0 K  T_nominal_specify=off  T_nominal_unit=K  T_nominal_value=1  Q_specify=off  Q_priority=None  Q=0 W  Q_nominal_specify=off  Q_nominal_unit=W  Q_nominal_value=1
  air-gap convection AGP to RTO : SimscapeCustomBlocks_lib/Convective Heat Transfer  area=A_RTO m^2  T_specify=off  T_priority=None  T=0 K  T_nominal_specify=off  T_nominal_unit=K  T_nominal_value=1  Q_specify=off  Q_priority=None  Q=0 W  Q_nominal_specify=off  Q_nominal_unit=W  Q_nominal_value=1
  air-gap convection AGP to SSL : SimscapeCustomBlocks_lib/Convective Heat Transfer  area=A_SSL m^2  T_specify=off  T_priority=None  T=0 K  T_nominal_specify=off  T_nominal_unit=K  T_nominal_value=1  Q_specify=off  Q_priority=None  Q=0 W  Q_nominal_specify=off  Q_nominal_unit=W  Q_nominal_value=1
  air-gap convection AGP to STO : SimscapeCustomBlocks_lib/Convective Heat Transfer  area=A_STO m^2  T_specify=off  T_priority=None  T=0 K  T_nominal_specify=off  T_nominal_unit=K  T_nominal_value=1  Q_specify=off  Q_priority=None  Q=0 W  Q_nominal_specify=off  Q_nominal_unit=W  Q_nominal_value=1
  inner air convection EC to inner air : SimscapeCustomBlocks_lib/Convective Heat Transfer  area=A_EC m^2  T_specify=off  T_priority=None  T=0 K  T_nominal_specify=off  T_nominal_unit=K  T_nominal_value=1  Q_specify=off  Q_priority=None  Q=0 W  Q_nominal_specify=off  Q_nominal_unit=W  Q_nominal_value=1
  inner air convection ER to inner air : SimscapeCustomBlocks_lib/Convective Heat Transfer  area=A_ER m^2  T_specify=off  T_priority=None  T=0 K  T_nominal_specify=off  T_nominal_unit=K  T_nominal_value=1  Q_specify=off  Q_priority=None  Q=0 W  Q_nominal_specify=off  Q_nominal_unit=W  Q_nominal_value=1
  inner air convection WH to inner air : SimscapeCustomBlocks_lib/Convective Heat Transfer  area=A_WH m^2  T_specify=off  T_priority=None  T=0 K  T_nominal_specify=off  T_nominal_unit=K  T_nominal_value=1  Q_specify=off  Q_priority=None  Q=0 W  Q_nominal_specify=off  Q_nominal_unit=W  Q_nominal_value=1
  pump active : Constant  Value=0
  pump inactive : Constant  Value=1000
  share of add losses in iron : Gain  Gain=0.5
  share of add losses in winding : Gain  Gain=0.5
  T_EMaschine_Wickelkopf [K] : Outport
  T_EMaschine_Kuehlmittel [K] : Outport  Port=2
  T_EMaschine_Wicklung [K] : Outport  Port=3
  T_EMaschine_Kurzschlussring [K] : Outport  Port=4
  T_EMaschine_Rotorstaebe [K] : Outport  Port=5
  wires:
  PS-Simulink Converter2/1 -> Scope/1
  share of add losses in iron/1 -> Sum1/2
  P_Verlust_EMaschine_Luftwiderstand [W]/1 -> Simulink-PS Converter20/1
  STO share of active iron/1 -> Simulink-PS Converter15/1
  HTC_Luftspalt [W*m^-2*K^-1]/1 -> Simulink-PS Converter6/1, Simulink-PS Converter7/1, Simulink-PS Converter8/1, Simulink-PS Converter9/1
  RTO share of active iron/1 -> Simulink-PS Converter18/1
  SYO share of active iron/1 -> Simulink-PS Converter17/1
  P_Verlust_EMaschine_Lager [W]/1 -> Simulink-PS Converter19/1
  P_Verlust_EMaschine_WirkZus [W]/1 -> share of add losses in iron/1, share of add losses in winding/1
  RYO share of active iron/1 -> Simulink-PS Converter16/1
  Sum1/1 -> STO share of active iron/1, RTO share of active iron/1, RYO share of active iron/1, SYO share of active iron/1
  P_Verlust_EMaschine_Ummagnet [W]/1 -> Sum1/1
  HTC_Kurzschlussring [W*m^-2*K^-1]/1 -> Simulink-PS Converter10/1
  HTC_Wickelkopf [W*m^-2*K^-1]/1 -> Simulink-PS Converter11/1
  HTC_Endcap [W*m^-2*K^-1]/1 -> Simulink-PS Converter12/1
  PS-Simulink Converter1/1 -> Aufteilung Wicklungsverluste + Temperaturabhängiger ohmscher Widerstand/5(T_EMaschine_Wickelkopf [K]), Delay/1, T_EMaschine_Wickelkopf [K]/1  "T_EMaschine_Wickelkopf [K]"
  PS-Simulink Converter4/1 -> T_EMaschine_Kuehlmittel [K]/1  "T_EMaschine_Kuehlmittel [K]"
  HTC with coolant pump active/1 -> Switch/1
  HTC with coolant pump inactive/1 -> Switch/3
  Switch/1 -> Simulink-PS Converter4/1
  pump active/1 -> Switch1/1
  pump inactive/1 -> Switch1/3
  Switch1/1 -> Simulink-PS Converter3/1
  Delay/1 -> Switch1/2, Switch/2
  PS-Simulink Converter3/1 -> Aufteilung Wicklungsverluste + Temperaturabhängiger ohmscher Widerstand/6(T_EMaschine_Wicklung [K]), T_EMaschine_Wicklung [K]/1  "T_EMaschine_Wicklung [K]"
  PS-Simulink Converter5/1 -> Aufteilung Wicklungsverluste + Temperaturabhängiger ohmscher Widerstand/4(T_EMaschine_Kurzschlussring [K]), T_EMaschine_Kurzschlussring [K]/1  "T_EMaschine_Kurzschlussring [K]"
  PS-Simulink Converter6/1 -> Aufteilung Wicklungsverluste + Temperaturabhängiger ohmscher Widerstand/3(T_EMaschine_Rotorstaebe [K]), T_EMaschine_Rotorstaebe [K]/1  "T_EMaschine_Rotorstaebe [K]"
  P_Verlust_EMaschine_Wicklung [W]/1 -> Aufteilung Wicklungsverluste + Temperaturabhängiger ohmscher Widerstand/1(P_Verlust_EMaschine_Wicklung [W])
  share of add losses in winding/1 -> Aufteilung Wicklungsverluste + Temperaturabhängiger ohmscher Widerstand/2(WirkZus-Verluste in Wicklung [W])
  Aufteilung Wicklungsverluste + Temperaturabhängiger ohmscher Widerstand/1(P_Verlust_EMaschine_Rotor_Nuten [W]) -> Simulink-PS Converter13/1
  Aufteilung Wicklungsverluste + Temperaturabhängiger ohmscher Widerstand/2(P_Verlust_EMaschine_Rotor_Kurzschlussring [W]) -> Simulink-PS Converter14/1
  Aufteilung Wicklungsverluste + Temperaturabhängiger ohmscher Widerstand/3(P_Verlust_EMaschine_Stator_Wickelkopf [W]) -> Simulink-PS Converter5/1
  Aufteilung Wicklungsverluste + Temperaturabhängiger ohmscher Widerstand/4(P_Verlust_EMaschine_Stator_Nuten [W]) -> Simulink-PS Converter1/1
  connections:
  PV_WH/LConn1 -- T_WH/LConn1 -- inner air convection WH to inner air/RConn1 -- C_WH/LConn1 -- R_toWH/RConn1
  R_toRSLTO/RConn1 -- C_RYO/LConn1 -- PV_RYO/LConn1 -- R_toSH/LConn1
  Simulink-PS Converter11/RConn1 -- inner air convection WH to inner air/LConn2
  R_toBR2/LConn1 -- R_toHO2/RConn1 -- C_EC/LConn1 -- inner air convection EC to inner air/RConn1
  Simulink-PS Converter9/RConn1 -- air-gap convection AGP to RTO/LConn2
  Simulink-PS Converter13/RConn1 -- PV_RSL/RConn1
  Thermal Reference7/LConn1 -- PV_SYO/RConn2
  C_SYO/LConn1 -- PV_SYO/LConn1 -- R_toHO/RConn1 -- R_toSSLTO/LConn1
  R_toSYO/LConn1 -- R_toSYO2/LConn1 -- R_toSSLTO/RConn1
  PV_WSL/LConn1 -- T_SSL/LConn1 -- C_SSL/LConn1 -- R_toSAGP/LConn1 -- R_toSYO/RConn1 -- R_toSTO/RConn1 -- R_toWH/LConn1
  PV_BR/LConn1 -- T_AGP/LConn1 -- R_toBR2/RConn1 -- R_toBR/RConn1
  R_toRAGP/RConn1 -- C_RSL/LConn1 -- T_RSL/LConn1 -- PV_RSL/LConn1 -- R_toER/LConn1 -- R_toRYO/LConn1 -- R_toRTO/RConn1
  air-gap convection AGP to STO/RConn1 -- R_toSAGP2/RConn1
  R_toRYO2/LConn1 -- PV_RTO/LConn1 -- C_RTO/LConn1 -- R_toRSL/LConn1 -- R_toRAGP2/RConn1
  Thermal Reference12/LConn1 -- PV_AGP/RConn2
  Thermal Reference8/LConn1 -- PV_STO/RConn2
  PV_SYO/RConn1 -- Simulink-PS Converter17/RConn1
  R_toRAGP/LConn1 -- air-gap convection AGP to RSL/RConn1
  R_toWC/LConn1 -- Convection HO to coolant/LConn1
  R_toRSL/RConn1 -- R_toRTO/LConn1
  Thermal Reference1/LConn1 -- PV_WSL/RConn2
  Thermal Reference5/LConn1 -- PV_RSL/RConn2
  Thermal Reference11/LConn1 -- PV_BR/RConn2
  Simulink-PS Converter20/RConn1 -- PV_AGP/RConn1
  Simulink-PS Converter10/RConn1 -- inner air convection ER to inner air/LConn2
  C_STO/LConn1 -- R_toSYO2/RConn1 -- R_toSAGP2/LConn1 -- R_toSSL/LConn1 -- PV_STO/LConn1
  R_toER/RConn1 -- T_ER/LConn1 -- inner air convection ER to inner air/RConn1 -- C_ER/LConn1 -- PV_ER/LConn1
  air-gap convection AGP to SSL/LConn1 -- air-gap convection AGP to STO/LConn1 -- PV_AGP/LConn1 -- air-gap convection AGP to RTO/LConn1 -- air-gap convection AGP to RSL/LConn1
  Thermal Reference9/LConn1 -- PV_RTO/RConn2
  R_toSH/RConn1 -- C_SH/LConn1 -- Solver Configuration1/RConn1 -- R_toBR/LConn1
  PV_STO/RConn1 -- Simulink-PS Converter15/RConn1
  PV_ER/RConn1 -- Simulink-PS Converter14/RConn1
  Thermal Reference10/LConn1 -- PV_RYO/RConn2
  Thermal Reference/LConn1 -- T_WH/RConn1
  Simulink-PS Converter6/RConn1 -- air-gap convection AGP to STO/LConn2
  PS-Simulink Converter2/LConn1 -- T_AGP/RConn2
  Simulink-PS Converter5/RConn1 -- PV_WH/RConn1
  Simulink-PS Converter12/RConn1 -- inner air convection EC to inner air/LConn2
  air-gap convection AGP to RSL/LConn2 -- Simulink-PS Converter8/RConn1
  PS-Simulink Converter1/LConn1 -- T_WH/RConn2
  Simulink-PS Converter19/RConn1 -- PV_BR/RConn1
  Thermal Reference6/LConn1 -- PV_ER/RConn2
  R_toSSL/RConn1 -- R_toSTO/LConn1
  Simulink-PS Converter7/RConn1 -- air-gap convection AGP to SSL/LConn2
  PV_RTO/RConn1 -- Simulink-PS Converter18/RConn1
  Thermal Reference3/LConn1 -- PV_WH/RConn2
  Thermal Reference4/LConn1 -- T_AGP/RConn1
  R_toSYO3/LConn1 -- R_toEC/LConn1 -- C_HO/LConn1 -- R_toWC/RConn1
  air-gap convection AGP to SSL/RConn1 -- R_toSAGP/RConn1
  R_toSYO3/RConn1 -- R_toHO/LConn1
  R_toRAGP2/LConn1 -- air-gap convection AGP to RTO/RConn1
  PV_WSL/RConn1 -- Simulink-PS Converter1/RConn1
  R_toHO2/LConn1 -- R_toEC/RConn1
  PV_RYO/RConn1 -- Simulink-PS Converter16/RConn1
  R_toRSLTO/LConn1 -- R_toRYO2/RConn1 -- R_toRYO/RConn1
  inner air convection EC to inner air/LConn1 -- inner air convection WH to inner air/LConn1 -- inner air convection ER to inner air/LConn1
  Konvektion Radiator an Umgebungsluft (keine Geschw.Abhängigkeit)/LConn1 -- C_WC water cooling pump active/LConn1 -- Variable Thermal Resistance/LConn1
  Umgebungslufttemperatur/LConn1 -- Konvektion Radiator an Umgebungsluft (keine Geschw.Abhängigkeit)/RConn1
  Thermal Reference2/LConn1 -- T_WC/RConn1
  PS-Simulink Converter4/LConn1 -- T_WC/RConn2
  Convection HO to coolant/LConn2 -- Simulink-PS Converter4/RConn1
  C_WC water cooling/LConn1 -- Variable Thermal Resistance/RConn1 -- Convection HO to coolant/RConn1 -- T_WC/LConn1
  Variable Thermal Resistance/LConn2 -- Simulink-PS Converter3/RConn1
  Thermal Reference14/LConn1 -- T_ER/RConn1
  T_ER/RConn2 -- PS-Simulink Converter5/LConn1
  Thermal Reference15/LConn1 -- T_RSL/RConn1
  T_RSL/RConn2 -- PS-Simulink Converter6/LConn1
  Thermal Reference13/LConn1 -- T_SSL/RConn1
  PS-Simulink Converter3/LConn1 -- T_SSL/RConn2

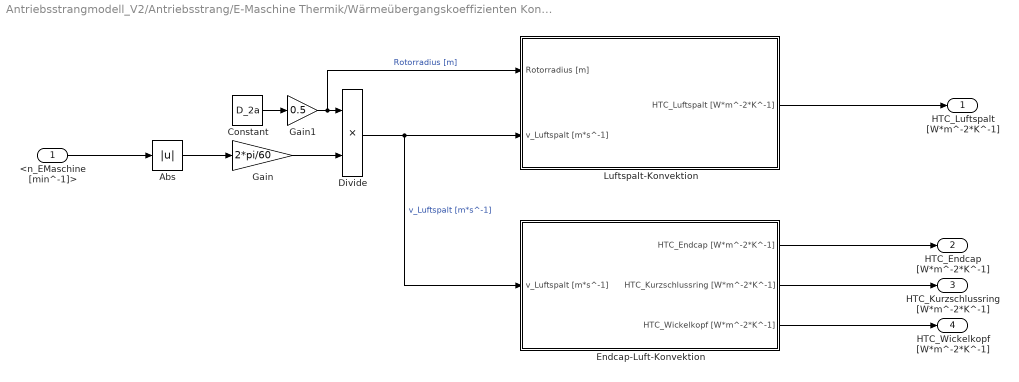
== system Antriebsstrangmodell_V2/Antriebsstrang/E-Maschine Thermik/Wärmeübergangskoeffizienten Konvektion Luftspalt und Endcap-Luft ==
  <n_EMaschine [min^-1]> : Inport
  Abs : Abs
  Constant : Constant  Value=D_2a
  Divide : Product  Inputs=**
  Endcap-Luft-Konvektion : Subsystem
  Gain : Gain  Gain=2*pi/60
  Gain1 : Gain  Gain=0.5
  Luftspalt-Konvektion : Subsystem
  HTC_Luftspalt [W*m^-2*K^-1] : Outport
  HTC_Endcap [W*m^-2*K^-1] : Outport  Port=2
  HTC_Kurzschlussring [W*m^-2*K^-1] : Outport  Port=3
  HTC_Wickelkopf [W*m^-2*K^-1] : Outport  Port=4
  wires:
  Gain1/1 -> Luftspalt-Konvektion/1(Rotorradius [m]), Divide/1  "Rotorradius [m]"
  <n_EMaschine [min^-1]>/1 -> Abs/1
  Constant/1 -> Gain1/1
  Abs/1 -> Gain/1
  Gain/1 -> Divide/2
  Divide/1 -> Endcap-Luft-Konvektion/1(v_Luftspalt [m*s^-1]), Luftspalt-Konvektion/2(v_Luftspalt [m*s^-1])  "v_Luftspalt [m*s^-1]"
  Luftspalt-Konvektion/1(HTC_Luftspalt [W*m^-2*K^-1]) -> HTC_Luftspalt [W*m^-2*K^-1]/1
  Endcap-Luft-Konvektion/1(HTC_Endcap [W*m^-2*K^-1]) -> HTC_Endcap [W*m^-2*K^-1]/1
  Endcap-Luft-Konvektion/2(HTC_Kurzschlussring [W*m^-2*K^-1]) -> HTC_Kurzschlussring [W*m^-2*K^-1]/1
  Endcap-Luft-Konvektion/3(HTC_Wickelkopf [W*m^-2*K^-1]) -> HTC_Wickelkopf [W*m^-2*K^-1]/1

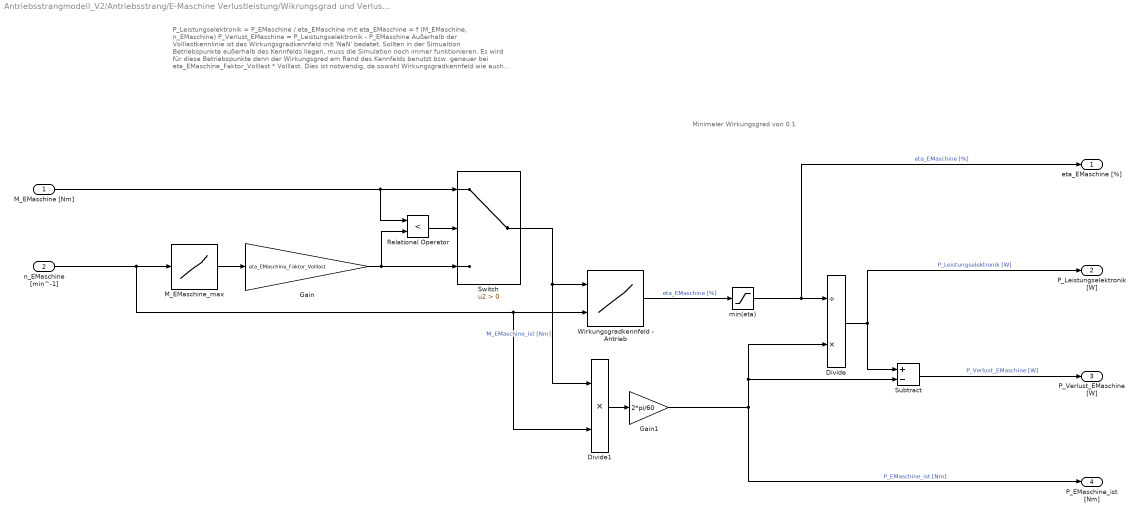
== system Antriebsstrangmodell_V2/Antriebsstrang/E-Maschine Verlustleistung/Wikrungsgrad und Verlustleistung - Antrieb ==
  note: Minimaler Wirkungsgrad von 0.1
  note: P_Leistungselektronik = P_EMaschine / eta_EMaschine
      |
      | mit eta_EMaschine = f (M_EMaschine, n_EMaschine)
      |
      | P_Verlust_EMaschine = P_Leistungselektronik - P_EMaschine
      |
      | Außerhalb der Volllastkennlinie ist das Wirkungsgradkennfeld mit 'NaN' bedatet. Sollten in der Simualtion Betriebspunkte außerhalb des Kennfelds liegen, muss die Simulation noch immer funktionieren. Es wird für diese Betriebspunkte dann der Wirkungsgrad am Rand des Kennfelds benutzt bzw. genauer bei eta_EMaschine_Faktor_Volllast * Volllast. Dies ist notwendig, da sowohl Wirkungsgradkennfeld wie auch Lookup Table nicht stetig sind und somit zwischen Stützstellen interpolieren müssen. Dies kann dazu führen, dass ein Wert, der auf der Volllastlinie sitzt, in 'NaN' im Wirkungsgradkennfeld resultiert. Um dies zu vermeiden, wird mit eta_EMaschine_Faktor_Volllast * Volllast gerechnet, wenn Betriebspunkte außerhalb des Kennfelds liegen, um 'NaN' Wirkungsgrade zu vermeiden. eta_EMaschine_Faktor_Volllast ist stark abh. von der Güte (Abstand der Stützstellen) des Wirkungsgradkennfeldes.
  M_EMaschine [Nm] : Inport
  n_EMaschine [min^-1] : Inport  Port=2
  Divide : Product  Inputs=/*
  Divide1 : Product  Inputs=**
  Gain : Gain  Gain=eta_EMaschine_Faktor_Volllast
  Gain1 : Gain  Gain=2*pi/60
  M_EMaschine_max : Lookup_n-D  NumberOfTableDimensions=1  BreakpointsForDimension1=M_EMaschine_max(1,:)  BeginIndexSearchUsingPreviousIndexResult=on  Table=M_EMaschine_max(2,:)  ExtrapMethod=Clip  UseLastTableValue=on  InternalRulePriority=Speed  RndMeth=Simplest  InputSameDT=on
  Relational Operator : RelationalOperator  Operator=<  OutDataTypeStr=boolean  RndMeth=Simplest
  Subtract : Sum  Inputs=+-
  Switch : Switch  Criteria=u2 > Threshold
  Wirkungsgradkennfeld - Antrieb : Lookup_n-D  BreakpointsForDimension1=eta_EMaschine_Break_M_EMaschine  BreakpointsForDimension2=eta_EMaschine_Break_n_EMaschine  BeginIndexSearchUsingPreviousIndexResult=on  Table=eta_EMaschine_Table  ExtrapMethod=Clip  UseLastTableValue=on  InternalRulePriority=Speed  RndMeth=Simplest  InputSameDT=on
  min(eta) : Saturate  UpperLimit=inf  LowerLimit=0.1
  eta_EMaschine [%] : Outport
  P_Leistungselektronik [W] : Outport  Port=2
  P_Verlust_EMaschine [W] : Outport  Port=3
  P_EMaschine_ist [Nm] : Outport  Port=4
  wires:
  Relational Operator/1 -> Switch/2
  Switch/1 -> Divide1/1, Wirkungsgradkennfeld - Antrieb/1  "M_EMaschine_ist [Nm]"
  Subtract/1 -> P_Verlust_EMaschine [W]/1  "P_Verlust_EMaschine [W]"
  n_EMaschine [min^-1]/1 -> Divide1/2, Wirkungsgradkennfeld - Antrieb/2, M_EMaschine_max/1
  Wirkungsgradkennfeld - Antrieb/1 -> min(eta)/1  "eta_EMaschine [%]"
  Gain/1 -> Relational Operator/2, Switch/3
  min(eta)/1 -> eta_EMaschine [%]/1, Divide/1  "eta_EMaschine [%]"
  M_EMaschine_max/1 -> Gain/1
  M_EMaschine [Nm]/1 -> Switch/1, Relational Operator/1
  Divide/1 -> P_Leistungselektronik [W]/1, Subtract/1  "P_Leistungselektronik [W]"
  Divide1/1 -> Gain1/1
  Gain1/1 -> P_EMaschine_ist [Nm]/1, Subtract/2, Divide/2  "P_EMaschine_ist [Nm]"

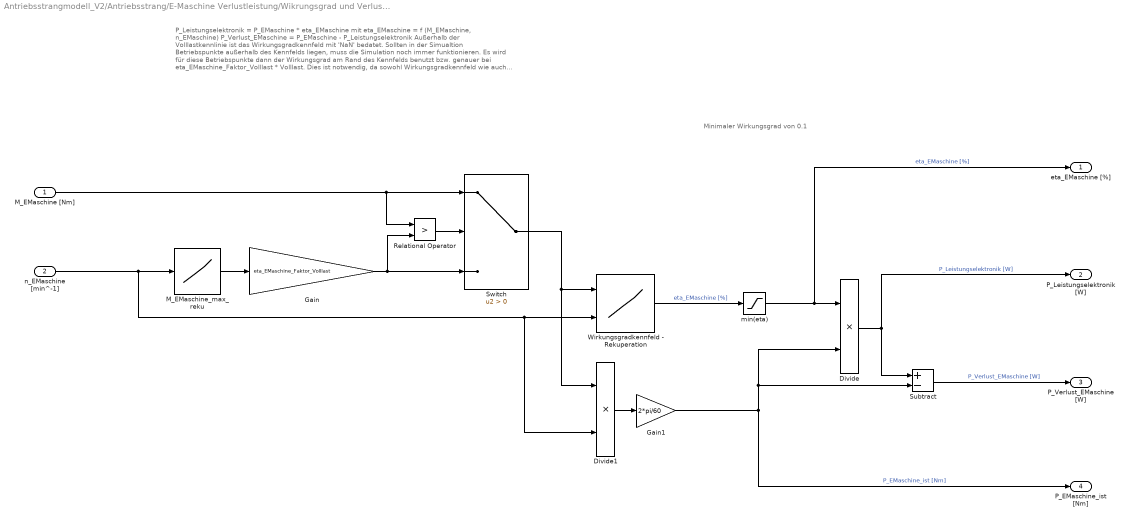
== system Antriebsstrangmodell_V2/Antriebsstrang/E-Maschine Verlustleistung/Wikrungsgrad und Verlustleistung - Rekuperation ==
  note: Minimaler Wirkungsgrad von 0.1
  note: P_Leistungselektronik = P_EMaschine * eta_EMaschine
      |
      | mit eta_EMaschine = f (M_EMaschine, n_EMaschine)
      |
      | P_Verlust_EMaschine = P_EMaschine - P_Leistungselektronik
      |
      | Außerhalb der Volllastkennlinie ist das Wirkungsgradkennfeld mit 'NaN' bedatet. Sollten in der Simualtion Betriebspunkte außerhalb des Kennfelds liegen, muss die Simulation noch immer funktionieren. Es wird für diese Betriebspunkte dann der Wirkungsgrad am Rand des Kennfelds benutzt bzw. genauer bei eta_EMaschine_Faktor_Volllast * Volllast. Dies ist notwendig, da sowohl Wirkungsgradkennfeld wie auch Lookup Table nicht stetig sind und somit zwischen Stützstellen interpolieren müssen. Dies kann dazu führen, dass ein Wert, der auf der Volllastlinie sitzt, in 'NaN' im Wirkungsgradkennfeld resultiert. Um dies zu vermeiden, wird mit eta_EMaschine_Faktor_Volllast * Volllast gerechnet, wenn Betriebspunkte außerhalb des Kennfelds liegen, um 'NaN' Wirkungsgrade zu vermeiden. eta_EMaschine_Faktor_Volllast ist stark abh. von der Güte (Abstand der Stützstellen) des Wirkungsgradkennfeldes.
  M_EMaschine [Nm] : Inport
  n_EMaschine [min^-1] : Inport  Port=2
  Divide : Product  Inputs=**
  Divide1 : Product  Inputs=**
  Gain : Gain  Gain=eta_EMaschine_Faktor_Volllast
  Gain1 : Gain  Gain=2*pi/60
  M_EMaschine_max_reku : Lookup_n-D  NumberOfTableDimensions=1  BreakpointsForDimension1=[-15,1700,2050,3400,4050,6100]  BeginIndexSearchUsingPreviousIndexResult=on  Table=[0.44,-52,-51,-37.5,-33,-27.25]  ExtrapMethod=Clip  UseLastTableValue=on  InternalRulePriority=Speed  RndMeth=Simplest  InputSameDT=on
  Relational Operator : RelationalOperator  Operator=>  OutDataTypeStr=boolean  RndMeth=Simplest
  Subtract : Sum  Inputs=+-
  Switch : Switch  Criteria=u2 > Threshold
  Wirkungsgradkennfeld - Rekuperation : Lookup_n-D  BreakpointsForDimension1=eta_EMaschine_Break_M_EMaschine_reku  BreakpointsForDimension2=eta_EMaschine_Break_n_EMaschine_reku  BeginIndexSearchUsingPreviousIndexResult=on  Table=eta_EMaschine_Table_reku  ExtrapMethod=Clip  UseLastTableValue=on  InternalRulePriority=Speed  RndMeth=Simplest  InputSameDT=on
  min(eta) : Saturate  UpperLimit=inf  LowerLimit=0.1
  eta_EMaschine [%] : Outport
  P_Leistungselektronik [W] : Outport  Port=2
  P_Verlust_EMaschine [W] : Outport  Port=3
  P_EMaschine_ist [Nm] : Outport  Port=4
  wires:
  Relational Operator/1 -> Switch/2
  Switch/1 -> Divide1/1, Wirkungsgradkennfeld - Rekuperation/1
  Subtract/1 -> P_Verlust_EMaschine [W]/1  "P_Verlust_EMaschine [W]"
  n_EMaschine [min^-1]/1 -> Divide1/2, Wirkungsgradkennfeld - Rekuperation/2, M_EMaschine_max_reku/1
  Wirkungsgradkennfeld - Rekuperation/1 -> min(eta)/1  "eta_EMaschine [%]"
  Gain/1 -> Relational Operator/2, Switch/3
  min(eta)/1 -> eta_EMaschine [%]/1, Divide/1  "eta_EMaschine [%]"
  M_EMaschine_max_reku/1 -> Gain/1
  M_EMaschine [Nm]/1 -> Switch/1, Relational Operator/1
  Divide/1 -> P_Leistungselektronik [W]/1, Subtract/1  "P_Leistungselektronik [W]"
  Divide1/1 -> Gain1/1
  Gain1/1 -> P_EMaschine_ist [Nm]/1, Subtract/2, Divide/2  "P_EMaschine_ist [Nm]"
